simulink model "DC_motor"  (R2023a)
settings: Solver=VariableStepAuto  StartTime=0.0  StopTime=0.2  RelTol=1e-3
values from neighbouring files (symbols this model uses):
  B = 0.00001    (= 1e-05)    [motor_model.m]
  C = pidtune(G, 'PID')    [motor_model.m]
  J = 0.000002    (= 2e-06)    [motor_model.m]
  K_e = 0.018    [motor_model.m]
  K_t = 0.018    [motor_model.m]
  L = 0.0005    [motor_model.m]
  R = 2.0    (= 2)    [motor_model.m]
libraries: slpidlib x1
settings Model: Creator=Faith Bamidele  LastModifiedBy=Faith Bamidele

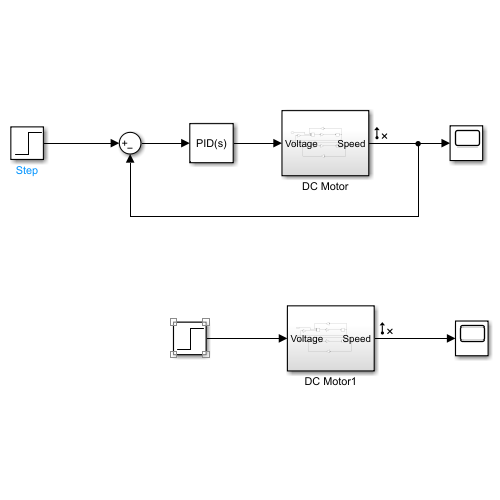
[thumbnail: Simulink's stored preview of the top-level diagram]
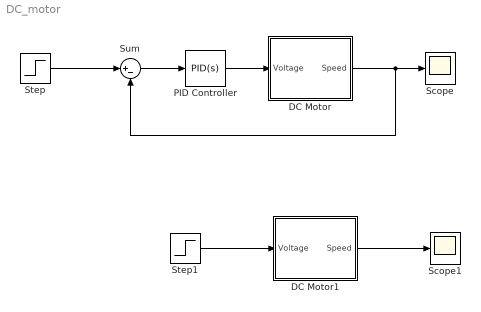
== system DC_motor ==
  DC Motor : Subsystem
  DC Motor1 : Subsystem
  PID Controller : slpidlib/PID Controller  Controller=PID  Form=Parallel  TimeDomain=Continuous-time  UseExternalTs=off  SampleTime=-1  IntegratorMethod=Forward Euler  FilterMethod=Forward Euler  ControllerParametersSource=internal  P=C.Kp  I=C.Ki  UseKiTs=off  D=C.Kd  N=100  UseFilter=on  TunerSelectOption=Transfer Function Based (PID Tuner App)  InitialConditionSource=internal  InitialConditionForIntegrator=0  InitialConditionForFilter=0  DifferentiatorICPrevScaledInput=0  ExternalReset=none  TrackingMode=off  Kt=1  LimitOutput=off  SatLimitsSource=internal  UpperSaturationLimit=inf  LowerSaturationLimit=-inf  LinearizeAsGain=on  AntiWindupMode=none  Kb=1  LimitIntegrator=off  UpperIntegratorSaturationLimit=inf  LowerIntegratorSaturationLimit=-inf  POutMin=[]  POutMax=[]  IOutMin=[]  IOutMax=[]  DOutMin=[]  DOutMax=[]  NOutMin=[]  NOutMax=[]  SumOutMin=[]  SumOutMax=[]  SaturationOutMin=[]  SaturationOutMax=[]  PParamMin=[]  PParamMax=[]  IParamMin=[]  IParamMax=[]  DParamMin=[]  DParamMax=[]  NParamMin=[]  NParamMax=[]  KbParamMin=[]  KbParamMax=[]  KtParamMin=[]  KtParamMax=[]  KbOutMin=[]  KbOutMax=[]  KtOutMin=[]  KtOutMax=[]  IntegratorOutMin=[]  IntegratorOutMax=[]  FilterOutMin=[]  FilterOutMax=[]  SumI1OutMin=[]  SumI1OutMax=[]  SumI2OutMin=[]  SumI2OutMax=[]  SumI3OutMin=[]  SumI3OutMax=[]  SumI4OutMin=[]  SumI4OutMax=[]  SumDOutMin=[]  SumDOutMax=[]  DifferentiatorOutMin=[]  DifferentiatorOutMax=[]  FilterDiffOutCoefMin=[]  FilterDiffOutCoefMax=[]  ReciprocalOutMin=[]  ReciprocalOutMax=[]  SumDenOutMin=[]  SumDenOutMax=[]  SumNumOutMin=[]  SumNumOutMax=[]  DivideOutMin=[]  DivideOutMax=[]  UdiffTsProdOutMin=[]  UdiffTsProdOutMax=[]  NTsProdOutMin=[]  NTsProdOutMax=[]  UintegralTsProdOutMin=[]  UintegralTsProdOutMax=[]  UngainTsProdOutMin=[]  UngainTsProdOutMax=[]  ClampingZeroOutDataTypeStr=Inherit: Inherit via back propagation  ClampingZeroOutMin=[]  ClampingZeroOutMax=[]  FilterDenConstantOutDataTypeStr=Inherit: Inherit via back propagation  FilterDenConstantOutMin=[]  FilterDenConstantOutMax=[]  PCopyOutDataTypeStr=Inherit: Inherit via back propagation  PCopyOutMin=[]  PCopyOutMax=[]  NCopyOutDataTypeStr=Inherit: Inherit via back propagation  NCopyOutMin=[]  NCopyOutMax=[]  IntegratorContinuousStateAttributes=''  IntegratorStateMustResolveToSignalObject=off  IntegratorRTWStateStorageClass=Auto  FilterContinuousStateAttributes=''  FilterStateMustResolveToSignalObject=off  FilterRTWStateStorageClass=Auto  ParallelPVariant=InternalParameters  IdealPVariant=Disabled  IVariant=InternalParameters  DVariant=InternalParameters  IntegratorVariant=Continuous  SatVariant=Disabled  AWVariant=Passthrough  PCopyVariant=Disabled  TRVariant=Disabled  FdbkBlocksVariant=Forward  IdealPFdbkVariant=Disabled  SatFdbkVariant=Disabled  DerivativeFilterVariant=ContFilter  NVariant=InternalParameters  NCopyVariant=Disabled  FilterICVariant=InternalICsFilter  IntegratorICVariant=InternalICs  ExternalResetVariant=Disabled  TRSumVariant=Passthrough  SumFdbkVariant=Disabled  SumVariant=Sum_PID  TsampFilterVariant=InternalTs  TsampNgainVariant=Passthrough  TsampIntegralVariant=Disabled_SignalSpec  ExternalSaturationOutDataTypeStr=Inherit: Same as second input
  Scope : Scope
  Scope1 : Scope
  Step : Step  SampleTime=0
  Step1 : Step  Time=0  SampleTime=0
  Sum : Sum  Inputs=|+-
  wires:
  DC Motor/1(Speed) -> Sum/2, Scope/1
  Sum/1 -> PID Controller/1
  PID Controller/1 -> DC Motor/1(Voltage)
  Step1/1 -> DC Motor1/1(Voltage)
  DC Motor1/1(Speed) -> Scope1/1
  Step/1 -> Sum/1

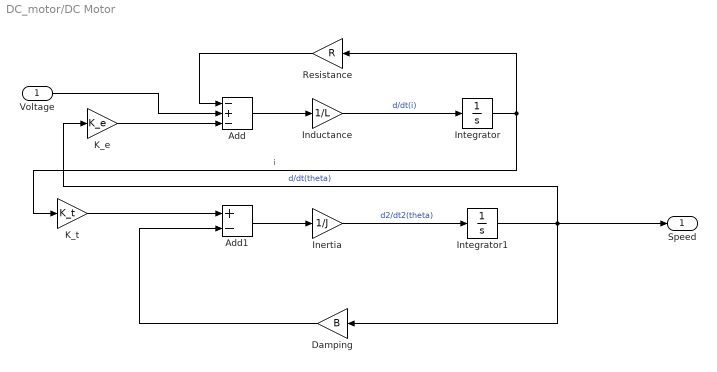
== system DC_motor/DC Motor ==
  Voltage : Inport
  Add : Sum  Inputs=-+-
  Add1 : Sum  Inputs=+-
  Damping : Gain  Gain=B
  Inductance : Gain  Gain=1/L
  Inertia : Gain  Gain=1/J
  Integrator : Integrator
  Integrator1 : Integrator
  K_e : Gain  Gain=K_e
  K_t : Gain  Gain=K_t
  Resistance : Gain  Gain=R
  Speed : Outport
  wires:
  Voltage/1 -> Add/2
  Inertia/1 -> Integrator1/1  "d2/dt2(theta)"
  Integrator1/1 -> Speed/1, K_e/1, Damping/1  "d/dt(theta)"
  Integrator/1 -> Resistance/1, K_t/1  "i"
  Inductance/1 -> Integrator/1  "d/dt(i)"
  K_t/1 -> Add1/1
  Add1/1 -> Inertia/1
  Damping/1 -> Add1/2
  Add/1 -> Inductance/1
  Resistance/1 -> Add/1
  K_e/1 -> Add/3

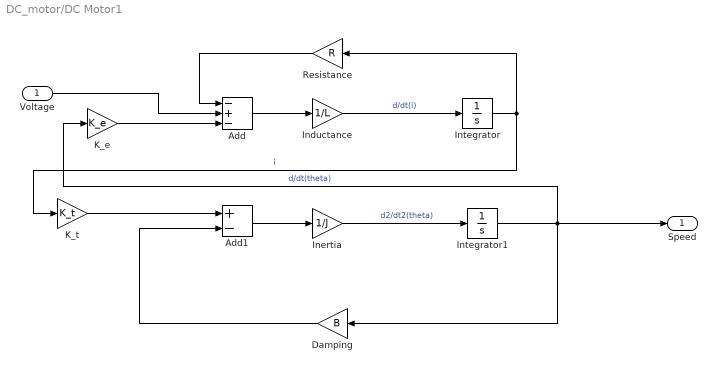
== system DC_motor/DC Motor1 ==
  Voltage : Inport
  Add : Sum  Inputs=-+-
  Add1 : Sum  Inputs=+-
  Damping : Gain  Gain=B
  Inductance : Gain  Gain=1/L
  Inertia : Gain  Gain=1/J
  Integrator : Integrator
  Integrator1 : Integrator
  K_e : Gain  Gain=K_e
  K_t : Gain  Gain=K_t
  Resistance : Gain  Gain=R
  Speed : Outport
  wires:
  Voltage/1 -> Add/2
  Inertia/1 -> Integrator1/1  "d2/dt2(theta)"
  Integrator1/1 -> Speed/1, K_e/1, Damping/1  "d/dt(theta)"
  Integrator/1 -> Resistance/1, K_t/1  "i"
  Inductance/1 -> Integrator/1  "d/dt(i)"
  K_t/1 -> Add1/1
  Add1/1 -> Inertia/1
  Damping/1 -> Add1/2
  Add/1 -> Inductance/1
  Resistance/1 -> Add/1
  K_e/1 -> Add/3
